simulink model "BMS_Model"  (R2024a)
settings: Solver=VariableStepAuto  StartTime=0.0  StopTime=10.0  RelTol=1e-3
libraries: simulink x1, hdlsllib x1
settings Model: Creator=saheb  LastModifiedBy=saheb

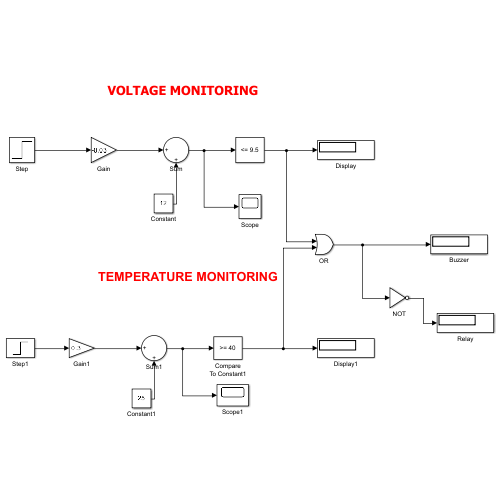
[thumbnail: Simulink's stored preview of the top-level diagram]
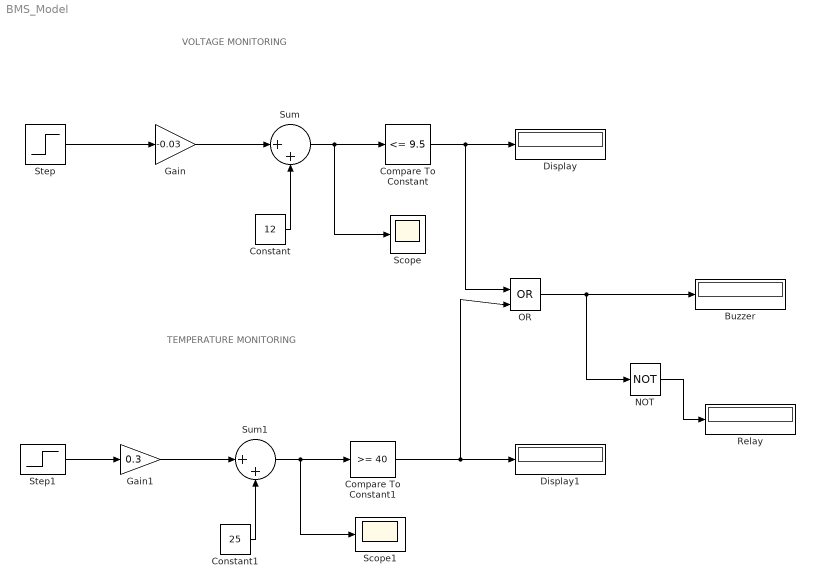
== system BMS_Model ==
  note: TEMPERATURE MONITORING
  note: VOLTAGE MONITORING
  Buzzer : Display
  Compare To Constant : simulink/Logic and Bit Operations/Compare To Constant  relop=<=  const=9.5  OutDataTypeStr=boolean
  Compare To Constant1 : hdlsllib/Logic and Bit Operations/Compare To Constant  relop=>=  const=40  OutDataTypeStr=boolean
  Constant : Constant  Value=12
  Constant1 : Constant  Value=25
  Display : Display
  Display1 : Display
  Gain : Gain  Gain=-0.03
  Gain1 : Gain  Gain=0.3
  NOT : Logic  Operator=NOT  IconShape=distinctive  AllPortsSameDT=off  OutDataTypeStr=boolean
  OR : Logic  Operator=OR  IconShape=distinctive  AllPortsSameDT=off  OutDataTypeStr=boolean
  Relay : Display
  Scope : Scope
  Scope1 : Scope
  Step : Step  SampleTime=0
  Step1 : Step  SampleTime=0
  Sum : Sum  Inputs=|++
  Sum1 : Sum  Inputs=|++
  wires:
  Step/1 -> Gain/1
  Gain/1 -> Sum/1
  Sum/1 -> Scope/1, Compare To Constant/1
  Step1/1 -> Gain1/1
  Gain1/1 -> Sum1/1
  Sum1/1 -> Scope1/1, Compare To Constant1/1
  Constant/1 -> Sum/2
  Compare To Constant/1 -> OR/1, Display/1
  Constant1/1 -> Sum1/2
  Compare To Constant1/1 -> OR/2, Display1/1
  OR/1 -> NOT/1, Buzzer/1
  NOT/1 -> Relay/1
